simulink model "fig10_67"  (Simulink 8.4)
settings: Solver=ode45  SolverMode=SingleTasking  StartTime=0.0  StopTime=100.0  RelTol=1e-5  AbsTol=1e-6
values from neighbouring files (symbols this model uses):
  A = [0    1.0000         0         0 ... (first row only)    [fig10_03.m]    (also in fig10_04.m; fig10_12.m; fig10_13.m; fig10_14.m)
  B = [0 ... (first row only)    [fig10_03.m]    (also in fig10_04.m; fig10_12.m; fig10_13.m; fig10_14.m)
  D = [0]    [fig10_03.m]    (also in fig10_04.m; fig10_12.m; fig10_13.m; fig10_14.m)
undefined symbols (not defined in the file or in its folder): C_center
libraries: simulink x1
CloseFcn:
  | ;slview('closediagram',bdroot);
settings Model: Creator=abbas  LastModifiedBy=abbas
settings DataIOCC: LimitDataPoints=off
settings OptimizationCC: BlockReduction=off  BooleanDataType=off  InitFltsAndDblsToZero=on
settings DebuggingCC: SaveWithParameterizedLinksMsg=none  SignalResolutionControl=TryResolveAllWithWarning  SolverPrmCheckMsg=none  MultiTaskDSMMsg=warning  MultiTaskCondExecSysMsg=none
settings HardwareCC: TargetUnknown=on
settings RTWCC: IncludeERTFirstTime=on
settings GRTTargetCC: TargetFcnLib=ansi_tfl_tmw.mat  ModelReferenceCompliant=off  CompOptLevelCompliant=off  MatFileLogging=off

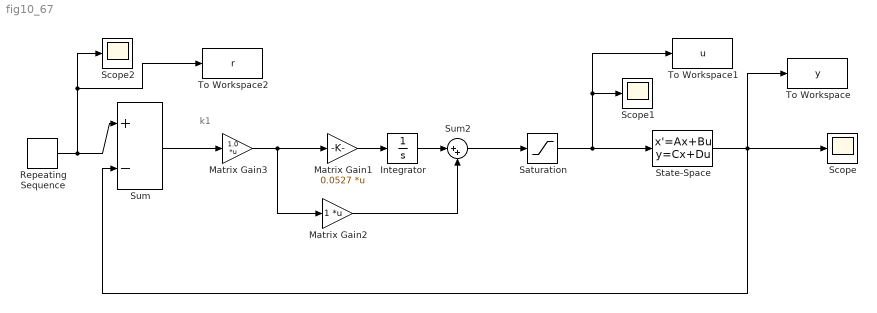
== system fig10_67 ==
  note: k1
  Integrator : Integrator
  Matrix Gain1 : Gain  Gain=0.0527  Multiplication=Matrix(K*u)  SaturateOnIntegerOverflow=on  OutDataTypeStr=Inherit: Same as input  ParamDataTypeStr=Inherit: Same as input
  Matrix Gain2 : Gain  Multiplication=Matrix(K*u)  SaturateOnIntegerOverflow=on  OutDataTypeStr=Inherit: Same as input  ParamDataTypeStr=Inherit: Same as input
  Matrix Gain3 : Gain  Gain=1.0  Multiplication=Matrix(K*u)  SaturateOnIntegerOverflow=on  OutDataTypeStr=Inherit: Same as input  ParamDataTypeStr=Inherit: Same as input
  Repeating Sequence : simulink/Sources/Repeating Sequence  rep_seq_t=[0:0.1:100]  rep_seq_y=[0:.1:25 25*ones(1,500) 0*ones(1,250)]
  Saturation : Saturate  UpperLimit=100  LowerLimit=-100
  Scope : Scope
      settings: TickLabels=on  TimeRange=100  YMin=0  YMax=100
  Scope1 : Scope
      settings: TickLabels=on
  Scope2 : Scope
      settings: TickLabels=on
  State-Space : StateSpace  A=A  B=B  C=C_center  D=D  X0=0
  Sum : Sum  Inputs=+-  SaturateOnIntegerOverflow=on  InputSameDT=on  OutDataTypeStr=Inherit: Same as first input
  Sum2 : Sum  Inputs=|++  SaturateOnIntegerOverflow=on  InputSameDT=on  OutDataTypeStr=Inherit: Same as first input
  To Workspace : ToWorkspace  VariableName=y  SampleTime=-1
  To Workspace1 : ToWorkspace  VariableName=u  SampleTime=-1
  To Workspace2 : ToWorkspace  VariableName=r  SampleTime=-1
  wires:
  Matrix Gain1/1 -> Integrator/1
  State-Space/1 -> Scope/1, Sum/2, To Workspace/1
  Matrix Gain2/1 -> Sum2/2
  Integrator/1 -> Sum2/1
  Sum2/1 -> Saturation/1
  Saturation/1 -> State-Space/1, Scope1/1, To Workspace1/1
  Sum/1 -> Matrix Gain3/1
  Matrix Gain3/1 -> Matrix Gain1/1, Matrix Gain2/1
  Repeating Sequence/1 -> Sum/1, Scope2/1, To Workspace2/1
